simulink model "data_logger"  (R2024a)
(part 2 of 2)

      | 				<Parameters>
      | 					<Parameter Name="Name">MAIN.fbRedCrane.fbStrokeToAngle.fMainAngle</Parameter>
      | 					<Parameter Name="SymbolName">MAIN.fbRedCrane.fbStrokeToAngle.fMainAngle</Parameter>
      | 					<Parameter Name="SymbolType">LREAL</Parameter>
      | 					<Parameter Name="SymbolGuid">{18071995-0000-0000-0000-00000000000E}</Parameter>
      | 					<Parameter Name="AmsNetId">128.39.200.164.1.1</Parameter>
      | 					<Parameter Name="Port">851</Parameter>
      | 					<Parameter Name="IndexGroup">#x0</Parameter>
      | 					<Parameter Name="IndexOffset">#x0</Parameter>
      | 					<Parameter Name="BitSize">64</Parameter>
      | 					<Parameter Name="InterpolationMode">3</Parameter>
      | 					<Parameter Name="ExtrapolationMode">0</Parameter>
      | 					<Parameter Name="SymbolInfo">0300400000000000000000000100000078000000D0070000E9FD00001600000000000000000000000000000000000000000000000000000000000000000000007800000001000000000000000000000008000000000000000500000081100000050000000000000000004C5245414C0000009519071800000000000000000000000E02000F06446973706C61794D696E56616C7565002D3130303030000F05446973706C61794D617856616C756500313030303000000000</Parameter>
      | 					<Parameter Name="TargetPlatform">1</Parameter>
      | 					<Parameter Name="SampleTime TC[100ns]">100000</Parameter>
      | 					<Parameter Name="SampleTime">100000</Parameter>
      | 					<Parameter Name="ReadViaNotification">True</Parameter>
      | 					<Parameter Name="Transmode">3</Parameter>
      | 					<Parameter Name="Timeout">1000</Parameter>
      | 					<Parameter Name="DelayTime">1000000</Parameter>
      | 					<Parameter Name="BufferSize">50</Parameter>
      | 					<Parameter Name="ByteSize">8</Parameter>
      | 					<Parameter Name="CodePage">65001</Parameter>
      | 				</Parameters>
      | 			</SymbolControlItem>
      | 			<SymbolControlItem GroupName="ADS Read" GroupDescription="Parameters for ADS Read command">
      | 				<Parameters>
      | 					<Parameter Name="Name">MAIN.fbRedCrane.fbStrokeToAngle.fKnuckleAngle</Parameter>
      | 					<Parameter Name="SymbolName">MAIN.fbRedCrane.fbStrokeToAngle.fKnuckleAngle</Parameter>
      | 					<Parameter Name="SymbolType">LREAL</Parameter>
      | 					<Parameter Name="SymbolGuid">{18071995-0000-0000-0000-00000000000E}</Parameter>
      | 					<Parameter Name="AmsNetId">128.39.200.164.1.1</Parameter>
      | 					<Parameter Name="Port">851</Parameter>
      | 					<Parameter Name="IndexGroup">#x0</Parameter>
      | 					<Parameter Name="IndexOffset">#x0</Parameter>
      | 					<Parameter Name="BitSize">64</Parameter>
      | 					<Parameter Name="InterpolationMode">3</Parameter>
      | 					<Parameter Name="ExtrapolationMode">0</Parameter>
      | 					<Parameter Name="SymbolInfo">0300400000000000000000000100000078000000D0070000E9FD00001600000000000000000000000000000000000000000000000000000000000000000000007800000001000000000000000000000008000000000000000500000081100000050000000000000000004C5245414C0000009519071800000000000000000000000E02000F06446973706C61794D696E56616C7565002D3130303030000F05446973706C61794D617856616C756500313030303000000000</Parameter>
      | 					<Parameter Name="TargetPlatform">1</Parameter>
      | 					<Parameter Name="SampleTime TC[100ns]">100000</Parameter>
      | 					<Parameter Name="SampleTime">100000</Parameter>
      | 					<Parameter Name="ReadViaNotification">True</Parameter>
      | 					<Parameter Name="Transmode">3</Parameter>
      | 					<Parameter Name="Timeout">1000</Parameter>
      | 					<Parameter Name="DelayTime">1000000</Parameter>
      | 					<Parameter Name="BufferSize">50</Parameter>
      | 					<Parameter Name="ByteSize">8</Parameter>
      | 					<Parameter Name="CodePage">65001</Parameter>
      | 				</Parameters>
      | 			</SymbolControlItem>
      | 			<SymbolControlItem GroupName="ADS Read" GroupDescription="Parameters for ADS Read command">
      | 				<Parameters>
      | 					<Parameter Name="Name">MAIN.fbRedCrane.fbInverceKinematics.fXRef</Parameter>
      | 					<Parameter Name="SymbolName">MAIN.fbRedCrane.fbInverceKinematics.fXRef</Parameter>
      | 					<Parameter Name="SymbolType">LREAL</Parameter>
      | 					<Parameter Name="SymbolGuid">{18071995-0000-0000-0000-00000000000E}</Parameter>
      | 					<Parameter Name="AmsNetId">128.39.200.164.1.1</Parameter>
      | 					<Parameter Name="Port">851</Parameter>
      | 					<Parameter Name="IndexGroup">#x0</Parameter>
      | 					<Parameter Name="IndexOffset">#x0</Parameter>
      | 					<Parameter Name="BitSize">64</Parameter>
      | 					<Parameter Name="InterpolationMode">3</Parameter>
      | 					<Parameter Name="ExtrapolationMode">0</Parameter>
      | 					<Parameter Name="SymbolInfo">0300400000000000000000000100000078000000D0070000E9FD00001600000000000000000000000000000000000000000000000000000000000000000000007800000001000000000000000000000008000000000000000500000081100000050000000000000000004C5245414C0000009519071800000000000000000000000E02000F06446973706C61794D696E56616C7565002D3130303030000F05446973706C61794D617856616C756500313030303000000000</Parameter>
      | 					<Parameter Name="TargetPlatform">1</Parameter>
      | 					<Parameter Name="SampleTime TC[100ns]">100000</Parameter>
      | 					<Parameter Name="SampleTime">100000</Parameter>
      | 					<Parameter Name="ReadViaNotification">True</Parameter>
      | 					<Parameter Name="Transmode">3</Parameter>
      | 					<Parameter Name="Timeout">1000</Parameter>
      | 					<Parameter Name="DelayTime">1000000</Parameter>
      | 					<Parameter Name="BufferSize">50</Parameter>
      | 					<Parameter Name="ByteSize">8</Parameter>
      | 					<Parameter Name="CodePage">65001</Parameter>
      | 				</Parameters>
      | 			</SymbolControlItem>
      | 			<SymbolControlItem GroupName="ADS Read" GroupDescription="Parameters for ADS Read command">
      | 				<Parameters>
      | 					<Parameter Name="Name">MAIN.fbRedCrane.fbInverceKinematics.fYRef</Parameter>
      | 					<Parameter Name="SymbolName">MAIN.fbRedCrane.fbInverceKinematics.fYRef</Parameter>
      | 					<Parameter Name="SymbolType">LREAL</Parameter>
      | 					<Parameter Name="SymbolGuid">{18071995-0000-0000-0000-00000000000E}</Parameter>
      | 					<Parameter Name="AmsNetId">128.39.200.164.1.1</Parameter>
      | 					<Parameter Name="Port">851</Parameter>
      | 					<Parameter Name="IndexGroup">#x0</Parameter>
      | 					<Parameter Name="IndexOffset">#x0</Parameter>
      | 					<Parameter Name="BitSize">64</Parameter>
      | 					<Parameter Name="InterpolationMode">3</Parameter>
      | 					<Parameter Name="ExtrapolationMode">0</Parameter>
      | 					<Parameter Name="SymbolInfo">0300400000000000000000000100000078000000D0070000E9FD00001600000000000000000000000000000000000000000000000000000000000000000000007800000001000000000000000000000008000000000000000500000081100000050000000000000000004C5245414C0000009519071800000000000000000000000E02000F06446973706C61794D696E56616C7565002D3130303030000F05446973706C61794D617856616C756500313030303000000000</Parameter>
      | 					<Parameter Name="TargetPlatform">1</Parameter>
      | 					<Parameter Name="SampleTime TC[100ns]">100000</Parameter>
      | 					<Parameter Name="SampleTime">100000</Parameter>
      | 					<Parameter Name="ReadViaNotification">True</Parameter>
      | 					<Parameter Name="Transmode">3</Parameter>
      | 					<Parameter Name="Timeout">1000</Parameter>
      | 					<Parameter Name="DelayTime">1000000</Parameter>
      | 					<Parameter Name="BufferSize">50</Parameter>
      | 					<Parameter Name="ByteSize">8</Parameter>
      | 					<Parameter Name="CodePage">65001</Parameter>
      | 				</Parameters>
      | 			</SymbolControlItem>
      | 			<SymbolControlItem GroupName="ADS Read" GroupDescription="Parameters for ADS Read command">
      | 				<Parameters>
      | 					<Parameter Name="Name">MAIN.fbRedCrane.fbInverceKinematics.fZRef</Parameter>
      | 					<Parameter Name="SymbolName">MAIN.fbRedCrane.fbInverceKinematics.fZRef</Parameter>
      | 					<Parameter Name="SymbolType">LREAL</Parameter>
      | 					<Parameter Name="SymbolGuid">{18071995-0000-0000-0000-00000000000E}</Parameter>
      | 					<Parameter Name="AmsNetId">128.39.200.164.1.1</Parameter>
      | 					<Parameter Name="Port">851</Parameter>
      | 					<Parameter Name="IndexGroup">#x0</Parameter>
      | 					<Parameter Name="IndexOffset">#x0</Parameter>
      | 					<Parameter Name="BitSize">64</Parameter>
      | 					<Parameter Name="InterpolationMode">3</Parameter>
      | 					<Parameter Name="ExtrapolationMode">0</Parameter>
      | 					<Parameter Name="SymbolInfo">0300400000000000000000000100000078000000D0070000E9FD00001600000000000000000000000000000000000000000000000000000000000000000000007800000001000000000000000000000008000000000000000500000081100000050000000000000000004C5245414C0000009519071800000000000000000000000E02000F06446973706C61794D696E56616C7565002D3130303030000F05446973706C61794D617856616C756500313030303000000000</Parameter>
      | 					<Parameter Name="TargetPlatform">1</Parameter>
      | 					<Parameter Name="SampleTime TC[100ns]">100000</Parameter>
      | 					<Parameter Name="SampleTime">100000</Parameter>
      | 					<Parameter Name="ReadViaNotification">True</Parameter>
      | 					<Parameter Name="Transmode">3</Parameter>
      | 					<Parameter Name="Timeout">1000</Parameter>
      | 					<Parameter Name="DelayTime">1000000</Parameter>
      | 					<Parameter Name="BufferSize">50</Parameter>
      | 					<Parameter Name="ByteSize">8</Parameter>
      | 					<Parameter Name="CodePage">65001</Parameter>
      | 				</Parameters>
      | 			</SymbolControlItem>
      | 			<SymbolControlItem GroupName="ADS Read" GroupDescription="Parameters for ADS Read command">
      | 				<Parameters>
      | 					<Parameter Name="Name">MAIN.fbRedCrane.fbForwardKinematics.fX</Parameter>
      | 					<Parameter Name="SymbolName">MAIN.fbRedCrane.fbForwardKinematics.fX</Parameter>
      | 					<Parameter Name="SymbolType">LREAL</Parameter>
      | 					<Parameter Name="SymbolGuid">{18071995-0000-0000-0000-00000000000E}</Parameter>
      | 					<Parameter Name="AmsNetId">128.39.200.164.1.1</Parameter>
      | 					<Parameter Name="Port">851</Parameter>
      | 					<Parameter Name="IndexGroup">#x0</Parameter>
      | 					<Parameter Name="IndexOffset">#x0</Parameter>
      | 					<Parameter Name="BitSize">64</Parameter>
      | 					<Parameter Name="InterpolationMode">3</Parameter>
      | 					<Parameter Name="ExtrapolationMode">0</Parameter>
      | 					<Parameter Name="SymbolInfo">0300400000000000000000000100000078000000D0070000E9FD00001600000000000000000000000000000000000000000000000000000000000000000000007800000001000000000000000000000008000000000000000500000081100000050000000000000000004C5245414C0000009519071800000000000000000000000E02000F06446973706C61794D696E56616C7565002D3130303030000F05446973706C61794D617856616C756500313030303000000000</Parameter>
      | 					<Parameter Name="TargetPlatform">1</Parameter>
      | 					<Parameter Name="SampleTime TC[100ns]">100000</Parameter>
      | 					<Parameter Name="SampleTime">100000</Parameter>
      | 					<Parameter Name="ReadViaNotification">True</Parameter>
      | 					<Parameter Name="Transmode">3</Parameter>
      | 					<Parameter Name="Timeout">1000</Parameter>
      | 					<Parameter Name="DelayTime">1000000</Parameter>
      | 					<Parameter Name="BufferSize">50</Parameter>
      | 					<Parameter Name="ByteSize">8</Parameter>
      | 					<Parameter Name="CodePage">65001</Parameter>
      | 				</Parameters>
      | 			</SymbolControlItem>
      | 			<SymbolControlItem GroupName="ADS Read" GroupDescription="Parameters for ADS Read command">
      | 				<Parameters>
      | 					<Parameter Name="Name">MAIN.fbRedCrane.fbForwardKinematics.fY</Parameter>
      | 					<Parameter Name="SymbolName">MAIN.fbRedCrane.fbForwardKinematics.fY</Parameter>
      | 					<Parameter Name="SymbolType">LREAL</Parameter>
      | 					<Parameter Name="SymbolGuid">{18071995-0000-0000-0000-00000000000E}</Parameter>
      | 					<Parameter Name="AmsNetId">128.39.200.164.1.1</Parameter>
      | 					<Parameter Name="Port">851</Parameter>
      | 					<Parameter Name="IndexGroup">#x0</Parameter>
      | 					<Parameter Name="IndexOffset">#x0</Parameter>
      | 					<Parameter Name="BitSize">64</Parameter>
      | 					<Parameter Name="InterpolationMode">3</Parameter>
      | 					<Parameter Name="ExtrapolationMode">0</Parameter>
      | 					<Parameter Name="SymbolInfo">0300400000000000000000000100000078000000D0070000E9FD00001600000000000000000000000000000000000000000000000000000000000000000000007800000001000000000000000000000008000000000000000500000081100000050000000000000000004C5245414C0000009519071800000000000000000000000E02000F06446973706C61794D696E56616C7565002D3130303030000F05446973706C61794D617856616C756500313030303000000000</Parameter>
      | 					<Parameter Name="TargetPlatform">1</Parameter>
      | 					<Parameter Name="SampleTime TC[100ns]">100000</Parameter>
      | 					<Parameter Name="SampleTime">100000</Parameter>
      | 					<Parameter Name="ReadViaNotification">True</Parameter>
      | 					<Parameter Name="Transmode">3</Parameter>
      | 					<Parameter Name="Timeout">1000</Parameter>
      | 					<Parameter Name="DelayTime">1000000</Parameter>
      | 					<Parameter Name="BufferSize">50</Parameter>
      | 					<Parameter Name="ByteSize">8</Parameter>
      | 					<Parameter Name="CodePage">65001</Parameter>
      | 				</Parameters>
      | 			</SymbolControlItem>
      | 			<SymbolControlItem GroupName="ADS Read" GroupDescription="Parameters for ADS Read command">
      | 				<Parameters>
      | 					<Parameter Name="Name">MAIN.fbRedCrane.fbForwardKinematics.fZ</Parameter>
      | 					<Parameter Name="SymbolName">MAIN.fbRedCrane.fbForwardKinematics.fZ</Parameter>
      | 					<Parameter Name="SymbolType">LREAL</Parameter>
      | 					<Parameter Name="SymbolGuid">{18071995-0000-0000-0000-00000000000E}</Parameter>
      | 					<Parameter Name="AmsNetId">128.39.200.164.1.1</Parameter>
      | 					<Parameter Name="Port">851</Parameter>
      | 					<Parameter Name="IndexGroup">#x0</Parameter>
      | 					<Parameter Name="IndexOffset">#x0</Parameter>
      | 					<Parameter Name="BitSize">64</Parameter>
      | 					<Parameter Name="InterpolationMode">3</Parameter>
      | 					<Parameter Name="ExtrapolationMode">0</Parameter>
      | 					<Parameter Name="SymbolInfo">0300400000000000000000000100000078000000D0070000E9FD00001600000000000000000000000000000000000000000000000000000000000000000000007800000001000000000000000000000008000000000000000500000081100000050000000000000000004C5245414C0000009519071800000000000000000000000E02000F06446973706C61794D696E56616C7565002D3130303030000F05446973706C61794D617856616C756500313030303000000000</Parameter>
      | 					<Parameter Name="TargetPlatform">1</Parameter>
      | 					<Parameter Name="SampleTime TC[100ns]">100000</Parameter>
      | 					<Parameter Name="SampleTime">100000</Parameter>
      | 					<Parameter Name="ReadViaNotification">True</Parameter>
      | 					<Parameter Name="Transmode">3</Parameter>
      | 					<Parameter Name="Timeout">1000</Parameter>
      | 					<Parameter Name="DelayTime">1000000</Parameter>
      | 					<Parameter Name="BufferSize">50</Parameter>
      | 					<Parameter Name="ByteSize">8</Parameter>
      | 					<Parameter Name="CodePage">65001</Parameter>
      | 				</Parameters>
      | 			</SymbolControlItem>
      | 			<SymbolControlItem GroupName="ADS Read" GroupDescription="Parameters for ADS Read command">
      | 				<Parameters>
      | 					<Parameter Name="Name">MAIN.fbRedCrane.fbSlewController_.fControlOutput</Parameter>
      | 					<Parameter Name="SymbolName">MAIN.fbRedCrane.fbSlewController_.fControlOutput</Parameter>
      | 					<Parameter Name="SymbolType">LREAL</Parameter>
      | 					<Parameter Name="SymbolGuid">{18071995-0000-0000-0000-00000000000E}</Parameter>
      | 					<Parameter Name="AmsNetId">128.39.200.164.1.1</Parameter>
      | 					<Parameter Name="Port">851</Parameter>
      | 					<Parameter Name="IndexGroup">#x0</Parameter>
      | 					<Parameter Name="IndexOffset">#x0</Parameter>
      | 					<Parameter Name="BitSize">64</Parameter>
      | 					<Parameter Name="InterpolationMode">3</Parameter>
      | 					<Parameter Name="ExtrapolationMode">0</Parameter>
      | 					<Parameter Name="SymbolInfo">0300400000000000000000000100000078000000D0070000E9FD00001600000000000000000000000000000000000000000000000000000000000000000000007800000001000000000000000000000008000000000000000500000081100000050000000000000000004C5245414C0000009519071800000000000000000000000E02000F06446973706C61794D696E56616C7565002D3130303030000F05446973706C61794D617856616C756500313030303000000000</Parameter>
      | 					<Parameter Name="TargetPlatform">1</Parameter>
      | 					<Parameter Name="SampleTime TC[100ns]">100000</Parameter>
      | 					<Parameter Name="SampleTime">100000</Parameter>
      | 					<Parameter Name="ReadViaNotification">True</Parameter>
      | 					<Parameter Name="Transmode">3</Parameter>
      | 					<Parameter Name="Timeout">1000</Parameter>
      | 					<Parameter Name="DelayTime">1000000</Parameter>
      | 					<Parameter Name="BufferSize">50</Parameter>
      | 					<Parameter Name="ByteSize">8</Parameter>
      | 					<Parameter Name="CodePage">65001</Parameter>
      | 				</Parameters>
      | 			</SymbolControlItem>
      | 			<SymbolControlItem GroupName="ADS Read" GroupDescription="Parameters for ADS Read command">
      | 				<Parameters>
      | 					<Parameter Name="Name">MAIN.fbRedCrane.fbSlewController_.fPosFeedback</Parameter>
      | 					<Parameter Name="SymbolName">MAIN.fbRedCrane.fbSlewController_.fPosFeedback</Parameter>
      | 					<Parameter Name="SymbolType">LREAL</Parameter>
      | 					<Parameter Name="SymbolGuid">{18071995-0000-0000-0000-00000000000E}</Parameter>
      | 					<Parameter Name="AmsNetId">128.39.200.164.1.1</Parameter>
      | 					<Parameter Name="Port">851</Parameter>
      | 					<Parameter Name="IndexGroup">#x0</Parameter>
      | 					<Parameter Name="IndexOffset">#x0</Parameter>
      | 					<Parameter Name="BitSize">64</Parameter>
      | 					<Parameter Name="InterpolationMode">3</Parameter>
      | 					<Parameter Name="ExtrapolationMode">0</Parameter>
      | 					<Parameter Name="SymbolInfo">0300400000000000000000000100000078000000D0070000E9FD00001600000000000000000000000000000000000000000000000000000000000000000000007800000001000000000000000000000008000000000000000500000081100000050000000000000000004C5245414C0000009519071800000000000000000000000E02000F06446973706C61794D696E56616C7565002D3130303030000F05446973706C61794D617856616C756500313030303000000000</Parameter>
      | 					<Parameter Name="TargetPlatform">1</Parameter>
      | 					<Parameter Name="SampleTime TC[100ns]">100000</Parameter>
      | 					<Parameter Name="SampleTime">100000</Parameter>
      | 					<Parameter Name="ReadViaNotification">True</Parameter>
      | 					<Parameter Name="Transmode">3</Parameter>
      | 					<Parameter Name="Timeout">1000</Parameter>
      | 					<Parameter Name="DelayTime">1000000</Parameter>
      | 					<Parameter Name="BufferSize">50</Parameter>
      | 					<Parameter Name="ByteSize">8</Parameter>
      | 					<Parameter Name="CodePage">65001</Parameter>
      | 				</Parameters>
      | 			</SymbolControlItem>
      | 			<SymbolControlItem GroupName="ADS Read" GroupDescription="Parameters for ADS Read command">
      | 				<Parameters>
      | 					<Parameter Name="Name">MAIN.fbRedCrane.fbSlewController_.fPosRef</Parameter>
      | 					<Parameter Name="SymbolName">MAIN.fbRedCrane.fbSlewController_.fPosRef</Parameter>
      | 					<Parameter Name="SymbolType">LREAL</Parameter>
      | 					<Parameter Name="SymbolGuid">{18071995-0000-0000-0000-00000000000E}</Parameter>
      | 					<Parameter Name="AmsNetId">128.39.200.164.1.1</Parameter>
      | 					<Parameter Name="Port">851</Parameter>
      | 					<Parameter Name="IndexGroup">#x0</Parameter>
      | 					<Parameter Name="IndexOffset">#x0</Parameter>
      | 					<Parameter Name="BitSize">64</Parameter>
      | 					<Parameter Name="InterpolationMode">3</Parameter>
      | 					<Parameter Name="ExtrapolationMode">0</Parameter>
      | 					<Parameter Name="SymbolInfo">0300400000000000000000000100000078000000D0070000E9FD00001600000000000000000000000000000000000000000000000000000000000000000000007800000001000000000000000000000008000000000000000500000081100000050000000000000000004C5245414C0000009519071800000000000000000000000E02000F06446973706C61794D696E56616C7565002D3130303030000F05446973706C61794D617856616C756500313030303000000000</Parameter>
      | 					<Parameter Name="TargetPlatform">1</Parameter>
      | 					<Parameter Name="SampleTime TC[100ns]">100000</Parameter>
      | 					<Parameter Name="SampleTime">100000</Parameter>
      | 					<Parameter Name="ReadViaNotification">True</Parameter>
      | 					<Parameter Name="Transmode">3</Parameter>
      | 					<Parameter Name="Timeout">1000</Parameter>
      | 					<Parameter Name="DelayTime">1000000</Parameter>
      | 					<Parameter Name="BufferSize">50</Parameter>
      | 					<Parameter Name="ByteSize">8</Parameter>
      | 					<Parameter Name="CodePage">65001</Parameter>
      | 				</Parameters>
      | 			</SymbolControlItem>
      | 			<SymbolControlItem GroupName="ADS Read" GroupDescription="Parameters for ADS Read command">
      | 				<Parameters>
      | 					<Parameter Name="Name">MAIN.fbRedCrane.fbSlewController_.fError</Parameter>
      | 					<Parameter Name="SymbolName">MAIN.fbRedCrane.fbSlewController_.fError</Parameter>
      | 					<Parameter Name="SymbolType">LREAL</Parameter>
      | 					<Parameter Name="SymbolGuid">{18071995-0000-0000-0000-00000000000E}</Parameter>
      | 					<Parameter Name="AmsNetId">128.39.200.164.1.1</Parameter>
      | 					<Parameter Name="Port">851</Parameter>
      | 					<Parameter Name="IndexGroup">#x0</Parameter>
      | 					<Parameter Name="IndexOffset">#x0</Parameter>
      | 					<Parameter Name="BitSize">64</Parameter>
      | 					<Parameter Name="InterpolationMode">3</Parameter>
      | 					<Parameter Name="ExtrapolationMode">0</Parameter>
      | 					<Parameter Name="SymbolInfo">0300400000000000000000000100000078000000D0070000E9FD00001600000000000000000000000000000000000000000000000000000000000000000000007800000001000000000000000000000008000000000000000500000081100000050000000000000000004C5245414C0000009519071800000000000000000000000E02000F06446973706C61794D696E56616C7565002D3130303030000F05446973706C61794D617856616C756500313030303000000000</Parameter>
      | 					<Parameter Name="TargetPlatform">1</Parameter>
      | 					<Parameter Name="SampleTime TC[100ns]">100000</Parameter>
      | 					<Parameter Name="SampleTime">100000</Parameter>
      | 					<Parameter Name="ReadViaNotification">True</Parameter>
      | 					<Parameter Name="Transmode">3</Parameter>
      | 					<Parameter Name="Timeout">1000</Parameter>
      | 					<Parameter Name="DelayTime">1000000</Parameter>
      | 					<Parameter Name="BufferSize">50</Parameter>
      | 					<Parameter Name="ByteSize">8</Parameter>
      | 					<Parameter Name="CodePage">65001</Parameter>
      | 				</Parameters>
      | 			</SymbolControlItem>
      | 			<SymbolControlItem GroupName="ADS Read" GroupDescription="Parameters for ADS Read command">
      | 				<Parameters>
      | 					<Parameter Name="Name">MAIN.fbRedCrane.fbPathPlanner.fbQuinticPathPlanner.bFinished</Parameter>
      | 					<Parameter Name="SymbolName">MAIN.fbRedCrane.fbPathPlanner.fbQuinticPathPlanner.bFinished</Parameter>
      | 					<Parameter Name="SymbolType">BOOL</Parameter>
      | 					<Parameter Name="SymbolGuid">{18071995-0000-0000-0000-000000000030}</Parameter>
      | 					<Parameter Name="AmsNetId">128.39.200.164.1.1</Parameter>
      | 					<Parameter Name="Port">851</Parameter>
      | 					<Parameter Name="IndexGroup">#x0</Parameter>
      | 					<Parameter Name="IndexOffset">#x0</Parameter>
      | 					<Parameter Name="BitSize">8</Parameter>
      | 					<Parameter Name="InterpolationMode">3</Parameter>
      | 					<Parameter Name="ExtrapolationMode">0</Parameter>
      | 					<Parameter Name="SymbolInfo">03004000000000000000000002000000E0000000D0070000E9FD0000160000000000000000000000000000000000000000000000000000000000000000000000700000000100000000000000000000000100000000000000110000008110000004000400000000000000424F4F4C004259544500009519071800000000000000000000003002000F01446973706C61794D696E56616C75650030000F01446973706C61794D617856616C756500310000700000000100000000000000000000000100000000000000110000008110000004000000000000000000425954450000009519071800000000000000000000000102000F01446973706C61794D696E56616C75650030000F04446973706C61794D617856616C75650023786666000000</Parameter>
      | 					<Parameter Name="TargetPlatform">1</Parameter>
      | 					<Parameter Name="SampleTime TC[100ns]">100000</Parameter>
      | 					<Parameter Name="SampleTime">100000</Parameter>
      | 					<Parameter Name="ReadViaNotification">True</Parameter>
      | 					<Parameter Name="Transmode">3</Parameter>
      | 					<Parameter Name="Timeout">1000</Parameter>
      | 					<Parameter Name="DelayTime">1000000</Parameter>
      | 					<Parameter Name="BufferSize">50</Parameter>
      | 					<Parameter Name="ByteSize">1</Parameter>
      | 					<Parameter Name="CodePage">65001</Parameter>
      | 				</Parameters>
      | 			</SymbolControlItem>
      | 			<SymbolControlItem GroupName="ADS Read" GroupDescription="Parameters for ADS Read command">
      | 				<Parameters>
      | 					<Parameter Name="Name">MAIN.fbRedCrane.fbPathPlanner.fXRef</Parameter>
      | 					<Parameter Name="SymbolName">MAIN.fbRedCrane.fbPathPlanner.fXRef</Parameter>
      | 					<Parameter Name="SymbolType">LREAL</Parameter>
      | 					<Parameter Name="SymbolGuid">{18071995-0000-0000-0000-00000000000E}</Parameter>
      | 					<Parameter Name="AmsNetId">128.39.200.164.1.1</Parameter>
      | 					<Parameter Name="Port">851</Parameter>
      | 					<Parameter Name="IndexGroup">#x0</Parameter>
      | 					<Parameter Name="IndexOffset">#x0</Parameter>
      | 					<Parameter Name="BitSize">64</Parameter>
      | 					<Parameter Name="InterpolationMode">3</Parameter>
      | 					<Parameter Name="ExtrapolationMode">0</Parameter>
      | 					<Parameter Name="SymbolInfo">0300400000000000000000000100000078000000D0070000E9FD00001600000000000000000000000000000000000000000000000000000000000000000000007800000001000000000000000000000008000000000000000500000081100000050000000000000000004C5245414C0000009519071800000000000000000000000E02000F06446973706C61794D696E56616C7565002D3130303030000F05446973706C61794D617856616C756500313030303000000000</Parameter>
      | 					<Parameter Name="TargetPlatform">1</Parameter>
      | 					<Parameter Name="SampleTime TC[100ns]">100000</Parameter>
      | 					<Parameter Name="SampleTime">100000</Parameter>
      | 					<Parameter Name="ReadViaNotification">True</Parameter>
      | 					<Parameter Name="Transmode">3</Parameter>
      | 					<Parameter Name="Timeout">1000</Parameter>
      | 					<Parameter Name="DelayTime">1000000</Parameter>
      | 					<Parameter Name="BufferSize">50</Parameter>
      | 					<Parameter Name="ByteSize">8</Parameter>
      | 					<Parameter Name="CodePage">65001</Parameter>
      | 				</Parameters>
      | 			</SymbolControlItem>
      | 			<SymbolControlItem GroupName="ADS Read" GroupDescription="Parameters for ADS Read command">
      | 				<Parameters>
      | 					<Parameter Name="Name">MAIN.fbRedCrane.fbPathPlanner.fYRef</Parameter>
      | 					<Parameter Name="SymbolName">MAIN.fbRedCrane.fbPathPlanner.fYRef</Parameter>
      | 					<Parameter Name="SymbolType">LREAL</Parameter>
      | 					<Parameter Name="SymbolGuid">{18071995-0000-0000-0000-00000000000E}</Parameter>
      | 					<Parameter Name="AmsNetId">128.39.200.164.1.1</Parameter>
      | 					<Parameter Name="Port">851</Parameter>
      | 					<Parameter Name="IndexGroup">#x0</Parameter>
      | 					<Parameter Name="IndexOffset">#x0</Parameter>
      | 					<Parameter Name="BitSize">64</Parameter>
      | 					<Parameter Name="InterpolationMode">3</Parameter>
      | 					<Parameter Name="ExtrapolationMode">0</Parameter>
      | 					<Parameter Name="SymbolInfo">0300400000000000000000000100000078000000D0070000E9FD00001600000000000000000000000000000000000000000000000000000000000000000000007800000001000000000000000000000008000000000000000500000081100000050000000000000000004C5245414C0000009519071800000000000000000000000E02000F06446973706C61794D696E56616C7565002D3130303030000F05446973706C61794D617856616C756500313030303000000000</Parameter>
      | 					<Parameter Name="TargetPlatform">1</Parameter>
      | 					<Parameter Name="SampleTime TC[100ns]">100000</Parameter>
      | 					<Parameter Name="SampleTime">100000</Parameter>
      | 					<Parameter Name="ReadViaNotification">True</Parameter>
      | 					<Parameter Name="Transmode">3</Parameter>
      | 					<Parameter Name="Timeout">1000</Parameter>
      | 					<Parameter Name="DelayTime">1000000</Parameter>
      | 					<Parameter Name="BufferSize">50</Parameter>
      | 					<Parameter Name="ByteSize">8</Parameter>
      | 					<Parameter Name="CodePage">65001</Parameter>
      | 				</Parameters>
      | 			</SymbolControlItem>
      | 			<SymbolControlItem GroupName="ADS Read" GroupDescription="Parameters for ADS Read command">
      | 				<Parameters>
      | 					<Parameter Name="Name">MAIN.fbRedCrane.fbPathPlanner.fZRef</Parameter>
      | 					<Parameter Name="SymbolName">MAIN.fbRedCrane.fbPathPlanner.fZRef</Parameter>
      | 					<Parameter Name="SymbolType">LREAL</Parameter>
      | 					<Parameter Name="SymbolGuid">{18071995-0000-0000-0000-00000000000E}</Parameter>
      | 					<Parameter Name="AmsNetId">128.39.200.164.1.1</Parameter>
      | 					<Parameter Name="Port">851</Parameter>
      | 					<Parameter Name="IndexGroup">#x0</Parameter>
      | 					<Parameter Name="IndexOffset">#x0</Parameter>
      | 					<Parameter Name="BitSize">64</Parameter>
      | 					<Parameter Name="InterpolationMode">3</Parameter>
      | 					<Parameter Name="ExtrapolationMode">0</Parameter>
      | 					<Parameter Name="SymbolInfo">0300400000000000000000000100000078000000D0070000E9FD00001600000000000000000000000000000000000000000000000000000000000000000000007800000001000000000000000000000008000000000000000500000081100000050000000000000000004C5245414C0000009519071800000000000000000000000E02000F06446973706C61794D696E56616C7565002D3130303030000F05446973706C61794D617856616C756500313030303000000000</Parameter>
      | 					<Parameter Name="TargetPlatform">1</Parameter>
      | 					<Parameter Name="SampleTime TC[100ns]">100000</Parameter>
      | 					<Parameter Name="SampleTime">100000</Parameter>
      | 					<Parameter Name="ReadViaNotification">True</Parameter>
      | 					<Parameter Name="Transmode">3</Parameter>
      | 					<Parameter Name="Timeout">1000</Parameter>
      | 					<Parameter Name="DelayTime">1000000</Parameter>
      | 					<Parameter Name="BufferSize">50</Parameter>
      | 					<Parameter Name="ByteSize">8</Parameter>
      | 					<Parameter Name="CodePage">65001</Parameter>
      | 				</Parameters>
      | 			</SymbolControlItem>
      | 			<SymbolControlItem GroupName="ADS Read" GroupDescription="Parameters for ADS Read command">
      | 				<Parameters>
      | 					<Parameter Name="Name">MAIN.fbRedCrane.fbForwardKinematics.fX_</Parameter>
      | 					<Parameter Name="SymbolName">MAIN.fbRedCrane.fbForwardKinematics.fX</Parameter>
      | 					<Parameter Name="SymbolType">LREAL</Parameter>
      | 					<Parameter Name="SymbolGuid">{18071995-0000-0000-0000-00000000000E}</Parameter>
      | 					<Parameter Name="AmsNetId">128.39.200.164.1.1</Parameter>
      | 					<Parameter Name="Port">851</Parameter>
      | 					<Parameter Name="IndexGroup">#x0</Parameter>
      | 					<Parameter Name="IndexOffset">#x0</Parameter>
      | 					<Parameter Name="BitSize">64</Parameter>
      | 					<Parameter Name="InterpolationMode">3</Parameter>
      | 					<Parameter Name="ExtrapolationMode">0</Parameter>
      | 					<Parameter Name="SymbolInfo">0300400000000000000000000100000078000000D0070000E9FD00001600000000000000000000000000000000000000000000000000000000000000000000007800000001000000000000000000000008000000000000000500000081100000050000000000000000004C5245414C0000009519071800000000000000000000000E02000F06446973706C61794D696E56616C7565002D3130303030000F05446973706C61794D617856616C756500313030303000000000</Parameter>
      | 					<Parameter Name="TargetPlatform">1</Parameter>
      | 					<Parameter Name="SampleTime TC[100ns]">100000</Parameter>
      | 					<Parameter Name="SampleTime">100000</Parameter>
      | 					<Parameter Name="ReadViaNotification">True</Parameter>
      | 					<Parameter Name="Transmode">3</Parameter>
      | 					<Parameter Name="Timeout">1000</Parameter>
      | 					<Parameter Name="DelayTime">1000000</Parameter>
      | 					<Parameter Name="BufferSize">50</Parameter>
      | 					<Parameter Name="ByteSize">8</Parameter>
      | 					<Parameter Name="CodePage">65001</Parameter>
      | 				</Parameters>
      | 			</SymbolControlItem>
      | 			<SymbolControlItem GroupName="ADS Read" GroupDescription="Parameters for ADS Read command">
      | 				<Parameters>
      | 					<Parameter Name="Name">MAIN.fbRedCrane.fbForwardKinematics.fY_</Parameter>
      | 					<Parameter Name="SymbolName">MAIN.fbRedCrane.fbForwardKinematics.fY</Parameter>
      | 					<Parameter Name="SymbolType">LREAL</Parameter>
      | 					<Parameter Name="SymbolGuid">{18071995-0000-0000-0000-00000000000E}</Parameter>
      | 					<Parameter Name="AmsNetId">128.39.200.164.1.1</Parameter>
      | 					<Parameter Name="Port">851</Parameter>
      | 					<Parameter Name="IndexGroup">#x0</Parameter>
      | 					<Parameter Name="IndexOffset">#x0</Parameter>
      | 					<Parameter Name="BitSize">64</Parameter>
      | 					<Parameter Name="InterpolationMode">3</Parameter>
      | 					<Parameter Name="ExtrapolationMode">0</Parameter>
      | 					<Parameter Name="SymbolInfo">0300400000000000000000000100000078000000D0070000E9FD00001600000000000000000000000000000000000000000000000000000000000000000000007800000001000000000000000000000008000000000000000500000081100000050000000000000000004C5245414C0000009519071800000000000000000000000E02000F06446973706C61794D696E56616C7565002D3130303030000F05446973706C61794D617856616C756500313030303000000000</Parameter>
      | 					<Parameter Name="TargetPlatform">1</Parameter>
      | 					<Parameter Name="SampleTime TC[100ns]">100000</Parameter>
      | 					<Parameter Name="SampleTime">100000</Parameter>
      | 					<Parameter Name="ReadViaNotification">True</Parameter>
      | 					<Parameter Name="Transmode">3</Parameter>
      | 					<Parameter Name="Timeout">1000</Parameter>
      | 					<Parameter Name="DelayTime">1000000</Parameter>
      | 					<Parameter Name="BufferSize">50</Parameter>
      | 					<Parameter Name="ByteSize">8</Parameter>
      | 					<Parameter Name="CodePage">65001</Parameter>
      | 				</Parameters>
      | 			</SymbolControlItem>
      | 			<SymbolControlItem GroupName="ADS Read" GroupDescription="Parameters for ADS Read command">
      | 				<Parameters>
      | 					<Parameter Name="Name">MAIN.fbRedCrane.fbForwardKinematics.fZ_</Parameter>
      | 					<Parameter Name="SymbolName">MAIN.fbRedCrane.fbForwardKinematics.fZ</Parameter>
      | 					<Parameter Name="SymbolType">LREAL</Parameter>
      | 					<Parameter Name="SymbolGuid">{18071995-0000-0000-0000-00000000000E}</Parameter>
      | 					<Parameter Name="AmsNetId">128.39.200.164.1.1</Parameter>
      | 					<Parameter Name="Port">851</Parameter>
      | 					<Parameter Name="IndexGroup">#x0</Parameter>
      | 					<Parameter Name="IndexOffset">#x0</Parameter>
      | 					<Parameter Name="BitSize">64</Parameter>
      | 					<Parameter Name="InterpolationMode">3</Parameter>
      | 					<Parameter Name="ExtrapolationMode">0</Parameter>
      | 					<Parameter Name="SymbolInfo">0300400000000000000000000100000078000000D0070000E9FD00001600000000000000000000000000000000000000000000000000000000000000000000007800000001000000000000000000000008000000000000000500000081100000050000000000000000004C5245414C0000009519071800000000000000000000000E02000F06446973706C61794D696E56616C7565002D3130303030000F05446973706C61794D617856616C756500313030303000000000</Parameter>
      | 					<Parameter Name="TargetPlatform">1</Parameter>
      | 					<Parameter Name="SampleTime TC[100ns]">100000</Parameter>
      | 					<Parameter Name="SampleTime">100000</Parameter>
      | 					<Parameter Name="ReadViaNotification">True</Parameter>
      | 					<Parameter Name="Transmode">3</Parameter>
      | 					<Parameter Name="Timeout">1000</Parameter>
      | 					<Parameter Name="DelayTime">1000000</Parameter>
      | 					<Parameter Name="BufferSize">50</Parameter>
      | 					<Parameter Name="ByteSize">8</Parameter>
      | 					<Parameter Name="CodePage">65001</Parameter>
      | 				</Parameters>
      | 			</SymbolControlItem>
      | 			<SymbolControlItem GroupName="ADS Read" GroupDescription="Parameters for ADS Read command">
      | 				<Parameters>
      | 					<Parameter Name="Name">MAIN.fbRedCrane.fbTelescopeController_.fPosFeedback</Parameter>
      | 					<Parameter Name="SymbolName">MAIN.fbRedCrane.fbTelescopeController_.fPosFeedback</Parameter>
      | 					<Parameter Name="SymbolType">LREAL</Parameter>
      | 					<Parameter Name="SymbolGuid">{18071995-0000-0000-0000-00000000000E}</Parameter>
      | 					<Parameter Name="AmsNetId">128.39.200.164.1.1</Parameter>
      | 					<Parameter Name="Port">851</Parameter>
      | 					<Parameter Name="IndexGroup">#x0</Parameter>
      | 					<Parameter Name="IndexOffset">#x0</Parameter>
      | 					<Parameter Name="BitSize">64</Parameter>
      | 					<Parameter Name="InterpolationMode">3</Parameter>
      | 					<Parameter Name="ExtrapolationMode">0</Parameter>
      | 					<Parameter Name="SymbolInfo">0300400000000000000000000100000078000000D0070000E9FD00001600000000000000000000000000000000000000000000000000000000000000000000007800000001000000000000000000000008000000000000000500000081100000050000000000000000004C5245414C0000009519071800000000000000000000000E02000F06446973706C61794D696E56616C7565002D3130303030000F05446973706C61794D617856616C756500313030303000000000</Parameter>
      | 					<Parameter Name="TargetPlatform">1</Parameter>
      | 					<Parameter Name="SampleTime TC[100ns]">100000</Parameter>
      | 					<Parameter Name="SampleTime">100000</Parameter>
      | 					<Parameter Name="ReadViaNotification">True</Parameter>
      | 					<Parameter Name="Transmode">3</Parameter>
      | 					<Parameter Name="Timeout">1000</Parameter>
      | 					<Parameter Name="DelayTime">1000000</Parameter>
      | 					<Parameter Name="BufferSize">50</Parameter>
      | 					<Parameter Name="ByteSize">8</Parameter>
      | 					<Parameter Name="CodePage">65001</Parameter>
      | 				</Parameters>
      | 			</SymbolControlItem>
      | 			<SymbolControlItem GroupName="ADS Read" GroupDescription="Parameters for ADS Read command">
      | 				<Parameters>
      | 					<Parameter Name="Name">MAIN.fbRedCrane.fbTelescopeController_.fPosRef</Parameter>
      | 					<Parameter Name="SymbolName">MAIN.fbRedCrane.fbTelescopeController_.fPosRef</Parameter>
      | 					<Parameter Name="SymbolType">LREAL</Parameter>
      | 					<Parameter Name="SymbolGuid">{18071995-0000-0000-0000-00000000000E}</Parameter>
      | 					<Parameter Name="AmsNetId">128.39.200.164.1.1</Parameter>
      | 					<Parameter Name="Port">851</Parameter>
      | 					<Parameter Name="IndexGroup">#x0</Parameter>
      | 					<Parameter Name="IndexOffset">#x0</Parameter>
      | 					<Parameter Name="BitSize">64</Parameter>
      | 					<Parameter Name="InterpolationMode">3</Parameter>
      | 					<Parameter Name="ExtrapolationMode">0</Parameter>
      | 					<Parameter Name="SymbolInfo">0300400000000000000000000100000078000000D0070000E9FD00001600000000000000000000000000000000000000000000000000000000000000000000007800000001000000000000000000000008000000000000000500000081100000050000000000000000004C5245414C0000009519071800000000000000000000000E02000F06446973706C61794D696E56616C7565002D3130303030000F05446973706C61794D617856616C756500313030303000000000</Parameter>
      | 					<Parameter Name="TargetPlatform">1</Parameter>
      | 					<Parameter Name="SampleTime TC[100ns]">100000</Parameter>
      | 					<Parameter Name="SampleTime">100000</Parameter>
      | 					<Parameter Name="ReadViaNotification">True</Parameter>
      | 					<Parameter Name="Transmode">3</Parameter>
      | 					<Parameter Name="Timeout">1000</Parameter>
      | 					<Parameter Name="DelayTime">1000000</Parameter>
      | 					<Parameter Name="BufferSize">50</Parameter>
      | 					<Parameter Name="ByteSize">8</Parameter>
      | 					<Parameter Name="CodePage">65001</Parameter>
      | 				</Parameters>
      | 			</SymbolControlItem>
      | 		</SymbolControlItems>
      | 	</Outputs>
      | </PortInfo>
      settings: SourceProductName=Beckhoff TwinCAT Interface
  TwinCAT Sync Clock : TcSimInterface/TwinCAT Sync Clock  ChangeRowColOrder=on  TraceMode=3  DirectFeedThrough=off  SignalLabels=3  PortLabels=2  ExpandBusObjDepth=on  SyncClockMode=Clock  SampleTime=-1
      settings: SourceProductName=Beckhoff TwinCAT Interface
  XY Graph : Record  FileSettingsInternal="{\"entries\":[{\"content\":{\"excelSettings\":{\"content\":{},\"type\":\"Streamout.ExcelSettings\"}},\"type\":\"Streamout.FileSettingStorage\",\"uuid\":\"\"}],\"packageUris\":[\"http:\\/\\/schema.mathworks.com\\/mf0\\/streamout_blocks\\/R2020a\"],\"version\":\"1.0\"}"  Layout=[1 1]  SignalsInternal="{\"entries\":[{\"content\":{\"signals\":[{\"content\":{\"blockPath\":[],\"dimensions\":[2],\"domain\":\"\",\"hasChildren\":true,\"lineColor\":\"#64d413\",\"lineWidth\":2,\"port\":1,\"sid\":[\"\"],\"signalID\":1,\"signalName\":\"Mux\"},\"type\":\"RecordBlkView.Signal\",\"uuid\":\"\"},{\"content\":{\"blockPath\":[],\"channel\":[1],\"dimensions\":[2],\"domain\":\"\",\"lineColor\":\"#ff13a6\",\"lineWidth\":2,\"parentID\":1,\"plots\":[ 1 ],\"port\":1,\"sid\":[\"\"],\"signalID\":2,\"signalName\":\"Mux\"},\"type\":\"RecordBlkView.Signal\",\"uuid\":\"\"},{\"content\":{\"blockPath\":[],\"dimensions\":[2],\"domain\":\"\",\"hasChildren\":true,\"lineColor\":\"#fe330a\",\"lineWidth\":2,\"port\":2,\"sid\":[\"\"],\"signalID\":3,\"signalName\":\"Mux1\"},\"type\":\"RecordBlkView.Signal\",\"uuid\":\"\"},{\"content\":{\"blockPath\":[],\"channel\":[1],\"dimensions\":[2],\"domain\":\"\",\"lineColor\":\"#7e2f8e\",\"lineWidth\":2,\"parentID\":3,\"plots\":[ 1 ],\"port\":2,\"sid\":[\"\"],\"signalID\":4,\"signalName\":\"Mux1\"},\"type\":\"RecordBlkView.Signal\",\"uuid\":\"\"},{\"content\":{\"blockPath\":[],\"channel\":[2],\"dimensions\":[2],\"domain\":\"\",\"lineColor\":\"#a2142f\",\"lineWidth\":2,\"parentID\":1,\"plots\":[ 1 ],\"port\":1,\"sid\":[\"\"],\"signalID\":5,\"signalName\":\"Mux\"},\"type\":\"RecordBlkView.Signal\",\"uuid\":\"\"},{\"content\":{\"blockPath\":[],\"channel\":[2],\"dimensions\":[2],\"domain\":\"\",\"lineColor\":\"#4dbeee\",\"lineWidth\":2,\"parentID\":3,\"plots\":[ 1 ],\"port\":2,\"sid\":[\"\"],\"signalID\":6,\"signalName\":\"Mux1\"},\"type\":\"RecordBlkView.Signal\",\"uuid\":\"\"}]},\"type\":\"RecordBlkView.InputSignals\",\"uuid\":\"\"}],\"packageUris\":[\"http:\\/\\/schema.mathworks.com\\/mf0\\/streamout_blocks\\/R2020a\"],\"version\":\"1.0\"}"  VisualizationBindings="{\"xyplotplugin\":{\"info\":[{\"series\":[],\"subplotID\":1}]}}"  CompatibilityTag=XY
  wires:
  Tc Symbol Interface/2 -> Scope/1  "MAIN.fbRedCrane.fbMainController_.fPosRef"
  Tc Symbol Interface/3 -> Scope/2  "MAIN.fbRedCrane.fbMainController_.fPosFeedback"
  Tc Symbol Interface/6 -> Scope1/1  "MAIN.fbRedCrane.fbKnuckleController_.fPosRef"
  Tc Symbol Interface/7 -> Scope1/2  "MAIN.fbRedCrane.fbKnuckleController_.fPosFeedback"
  Tc Symbol Interface/4 -> Scope2/1  "MAIN.fbRedCrane.fbMainController_.fControlOutput"
  Tc Symbol Interface/8 -> Scope2/2  "MAIN.fbRedCrane.fbKnuckleController_.fControlOutput"
  Tc Symbol Interface/9 -> Radians to Degrees/1  "MAIN.fbRedCrane.fbStrokeToAngle.fMainAngle"
  Tc Symbol Interface/10 -> Radians to Degrees1/1  "MAIN.fbRedCrane.fbStrokeToAngle.fKnuckleAngle"
  Radians to Degrees/1 -> Scope3/1  "fMainAngle"
  Radians to Degrees1/1 -> Scope3/2  "fKnuckleAngle"
  Constant/1 -> Tc Symbol Interface/1  "MAIN.fbRedCrane.fbMainController_.fKPPos"
  Constant4/1 -> Tc Symbol Interface/2  "MAIN.fbRedCrane.fbMainController_.fKPNeg"
  Constant1/1 -> Tc Symbol Interface/3  "MAIN.fbRedCrane.fbMainController_.fKffPos"
  Constant5/1 -> Tc Symbol Interface/4  "MAIN.fbRedCrane.fbMainController_.fKffNeg"
  Constant2/1 -> Tc Symbol Interface/5  "MAIN.fbRedCrane.fbKnuckleController_.fKPPos"
  Constant6/1 -> Tc Symbol Interface/6  "MAIN.fbRedCrane.fbKnuckleController_.fKPNeg"
  Constant3/1 -> Tc Symbol Interface/7  "MAIN.fbRedCrane.fbKnuckleController_.fKffPos"
  Constant7/1 -> Tc Symbol Interface/8  "MAIN.fbRedCrane.fbKnuckleController_.fKffNeg"
  Mux/1 -> XY Graph/1
  Mux1/1 -> XY Graph/2
  Tc Symbol Interface/11 -> Mux/1  "MAIN.fbRedCrane.fbInverceKinematics.fXRef"
  Tc Symbol Interface/14 -> Mux/2  "MAIN.fbRedCrane.fbForwardKinematics.fX"
  Tc Symbol Interface/13 -> Mux1/1  "MAIN.fbRedCrane.fbInverceKinematics.fZRef"
  Tc Symbol Interface/16 -> Mux1/2  "MAIN.fbRedCrane.fbForwardKinematics.fZ"
  Constant8/1 -> Tc Symbol Interface/9  "MAIN.fbRedCrane.fbSlewController_.fKPPos"
  Constant10/1 -> Tc Symbol Interface/10  "MAIN.fbRedCrane.fbSlewController_.fKPNeg"
  Constant9/1 -> Tc Symbol Interface/11  "MAIN.fbRedCrane.fbSlewController_.fKffPos"
  Constant11/1 -> Tc Symbol Interface/12  "MAIN.fbRedCrane.fbSlewController_.fKffNeg"
  Constant12/1 -> Cast To Double/1
  Cast To Double/1 -> Tc Symbol Interface/13  "MAIN.fbRedCrane.fbPathPlanner.nPointSetNumber"
  Constant13/1 -> Tc Symbol Interface/14  "MAIN.fbRedCrane.fbPathPlanner.wayPoint1"
  Constant14/1 -> Tc Symbol Interface/15  "MAIN.fbRedCrane.fbPathPlanner.wayPoint2"
  Constant16/1 -> Tc Symbol Interface/16  "MAIN.fbRedCrane.fbPathPlanner.wayPoint3"
  Constant15/1 -> Tc Symbol Interface/17  "MAIN.fbRedCrane.fbPathPlanner.wayPoint4"
  Constant17/1 -> Tc Symbol Interface/18  "MAIN.fbRedCrane.fbPathPlanner.fVmax"
  Tc Symbol Interface/22 -> Scope5/1  "MAIN.fbRedCrane.fbPathPlanner.fXRef"
  Tc Symbol Interface/25 -> Scope5/2  "MAIN.fbRedCrane.fbForwardKinematics.fX_"
  Tc Symbol Interface/23 -> Scope6/1  "MAIN.fbRedCrane.fbPathPlanner.fYRef"
  Tc Symbol Interface/26 -> Scope6/2  "MAIN.fbRedCrane.fbForwardKinematics.fY_"
  Tc Symbol Interface/24 -> Scope4/1  "MAIN.fbRedCrane.fbPathPlanner.fZRef"
  Tc Symbol Interface/27 -> Scope4/2  "MAIN.fbRedCrane.fbForwardKinematics.fZ_"
  Tc Symbol Interface/21 -> Scope7/1  "MAIN.fbRedCrane.fbPathPlanner.fbQuinticPathPlanner.bFinished"
  Constant18/1 -> Tc Symbol Interface/19  "MAIN.fbRedCrane.fbTelescopeController_.fKPNeg"
  Constant19/1 -> Tc Symbol Interface/20  "MAIN.fbRedCrane.fbTelescopeController_.fKPPos"
  Tc Symbol Interface/28 -> Scope8/1  "MAIN.fbRedCrane.fbTelescopeController_.fPosFeedback"
  Tc Symbol Interface/29 -> Scope8/2  "MAIN.fbRedCrane.fbTelescopeController_.fPosRef"
